simulink subsystem "HEVP3"  (R2024b)
settings: Solver=VariableStepAuto  StartTime=0.0  StopTime=10.0  RelTol=1e-3
undefined symbols (not defined in the file): Diff, Eng, Lock, PlntDriveshftDamp, PlntDriveshftStiff, PlntTransEffTempBpt, PlntTransGearRatioVect, Trans, up
libraries: autolibsharedcoupling x2, autolibsharedtransfixedgear x1, autolibtrqconv x1
settings Model: ModifiedByFormat=The MathWorks, Inc.  Creator=The MathWorks, Inc.  LastModifiedBy=The MathWorks, Inc.
settings SolverCC: MaxZcPerStep=1
settings DebuggingCC: UnconnectedInputMsg=warning  UnconnectedOutputMsg=warning  UnconnectedLineMsg=warning
settings ModelReferenceCC: EnableRefExpFcnMdlSchedulingChecks=on
settings RTWCC: GPUComputeCapability=3.5  DLArmComputeVersion=19.05

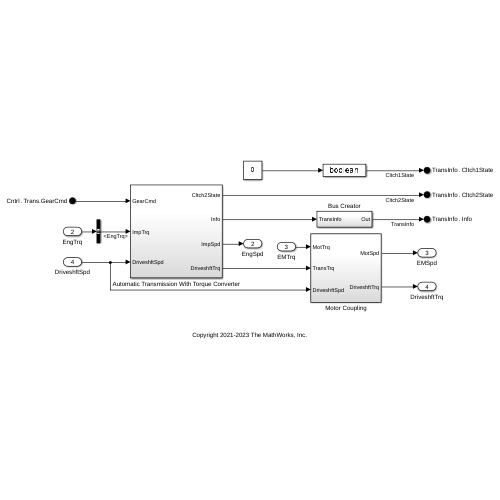
[thumbnail: Simulink's stored preview of the top-level diagram]
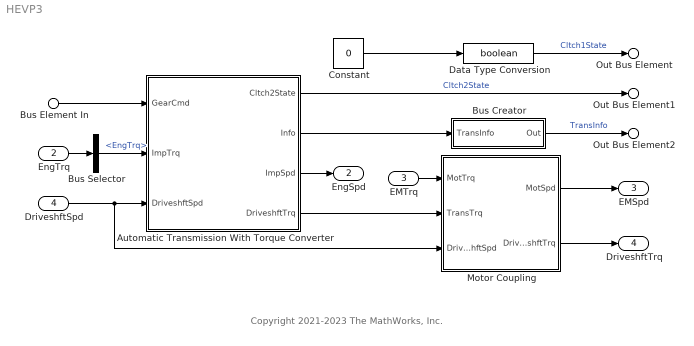
== system HEVP3 ==
  note: Copyright 2021-2023 The MathWorks, Inc.
  Bus Element In : Inport  PortName=Cntrl  Element=Trans.GearCmd
  EngTrq : Inport  Port=2
  EMTrq : Inport  Port=3
  DriveshftSpd : Inport  Port=4
  Automatic Transmission With Torque Converter : Subsystem  VariantControl=1
  Bus Selector : BusSelector  OutputSignals=EngTrq
  Bus Creator : Subsystem
  Constant : Constant  Value=0  SampleTime=-1
  Data Type Conversion : DataTypeConversion  OutDataTypeStr=boolean  SaturateOnIntegerOverflow=off  RndMeth=Floor
  Motor Coupling : Subsystem
  Out Bus Element : Outport  PortName=TransInfo  Element=Cltch1State
  Out Bus Element1 : Outport  PortName=TransInfo  Element=Cltch2State
  Out Bus Element2 : Outport  PortName=TransInfo  Element=Info
  EngSpd : Outport  Port=2  VectorParamsAs1DForOutWhenUnconnected=off  BusOutputAsStruct=on
  EMSpd : Outport  Port=3  VectorParamsAs1DForOutWhenUnconnected=off  BusOutputAsStruct=on
  DriveshftTrq : Outport  Port=4  VectorParamsAs1DForOutWhenUnconnected=off
  wires:
  Motor Coupling/1(MotSpd) -> EMSpd/1
  Bus Element In/1 -> Automatic Transmission With Torque Converter/1(GearCmd)
  EngTrq/1 -> Bus Selector/1
  EMTrq/1 -> Motor Coupling/1(MotTrq)
  Automatic Transmission With Torque Converter/3(ImpSpd) -> EngSpd/1
  DriveshftSpd/1 -> Automatic Transmission With Torque Converter/3(DriveshftSpd), Motor Coupling/3(DriveshftSpd)
  Automatic Transmission With Torque Converter/4(DriveshftTrq) -> Motor Coupling/2(TransTrq)
  Motor Coupling/2(DriveshftTrq) -> DriveshftTrq/1
  Automatic Transmission With Torque Converter/1(Cltch2State) -> Out Bus Element1/1  "Cltch2State"
  Data Type Conversion/1 -> Out Bus Element/1  "Cltch1State"
  Constant/1 -> Data Type Conversion/1
  Bus Selector/1 -> Automatic Transmission With Torque Converter/2(ImpTrq)  "<EngTrq>"
  Bus Creator/1(Out) -> Out Bus Element2/1  "TransInfo"
  Automatic Transmission With Torque Converter/2(Info) -> Bus Creator/1(TransInfo)

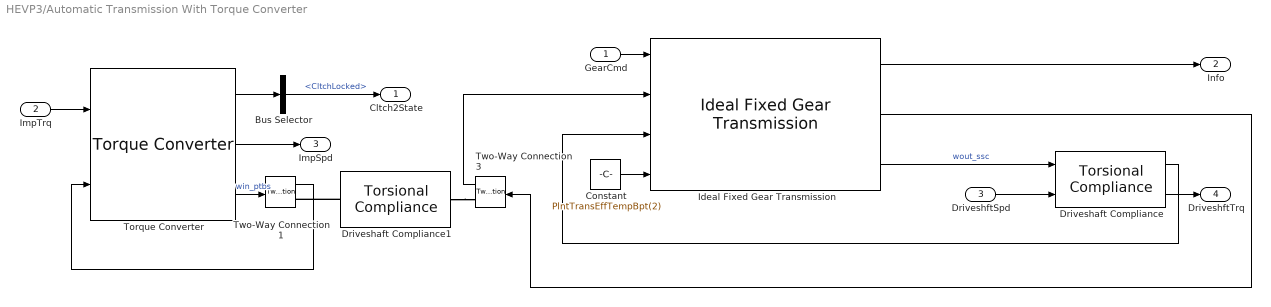
== system HEVP3/Automatic Transmission With Torque Converter ==
  GearCmd : Inport
  ImpTrq : Inport  Port=2
  DriveshftSpd : Inport  Port=3
  Bus Selector : BusSelector  OutputSignals=Cltch.CltchLocked
  Constant : Constant  Value=PlntTransEffTempBpt(2)  SampleTime=-1
  Driveshaft Compliance : autolibsharedcoupling/Torsional Compliance  port_config=Simulink  extInfo=off  k=PlntDriveshftStiff  b=PlntDriveshftDamp  theta_o=PlntDriveshftInitDeflect  domega_o=PlntDriveshftInitVel  omega_c=PlntDriveshftDampCutoffFreq  blkID=0  aMode=1
  Driveshaft Compliance1 : autolibsharedcoupling/Torsional Compliance  port_config=Two-way connection  extInfo=off  k=PlntDriveshftStiff  b=PlntDriveshftDamp  theta_o=PlntDriveshftInitDeflect  domega_o=PlntDriveshftInitVel  omega_c=PlntDriveshftDampCutoffFreq  blkID=0  aMode=1
  Ideal Fixed Gear Transmission : autolibsharedtransfixedgear/Ideal Fixed Gear Transmission  VariantControl=0  TransEffModelPopup=Gear, input torque, input speed, and temperature  gearInterp=Linear point-slope  G=PlntTransGearNumVect  Trq_bpts=PlntTransEffTrqBpt  omega_bpts=PlntTransEffSpdBpt  Temp_bpts=PlntTransEffTempBpt  N=PlntTransGearRatioVect  Jout=PlntTransInertiaVect  bout=PlntTransDampVect  eta=PlntTransEffVect  eta_tbl=PlntTransEffTbl  G_o=PlntTransInitGear  omega_o=PlntTransInitOutVel  omegaN_o=PlntTransInitNtrlInVel  tau_s=PlntTransShftTimeCnst  maxAbsSpd=5e3  aMode=6
  Torque Converter : autolibtrqconv/Torque Converter  TCType=Lock-up  port_config=Simulink  Ji=PlntTrqConvrtrImpInertia  bi=PlntTrqConvrtrImpDamp  Jt=PlntTrqConvrtrTurbInertia  bt=PlntTrqConvrtrTurbDamp  omegai_o=PlntTrqConvrtrImpInitVel  omegat_o=PlntTrqConvrtrTurbInitVel  phi=PlntTrqConvrtrSpdRatioVect  KType=Input speed / sqrt(input torque)  psi=PlntTrqConvrtrCapVect  zeta=PlntTrqConvrtrTrqRatioVect  tauTC=PlntTrqConvrtrTimeCnst  InterpMethod=Linear  Reff=PlntTrqConvrtrCltchRadius  mus=PlntTrqConvrtrCltchStatFric  muk=PlntTrqConvrtrCltchKinFric  ClutchLocked=off  philu=PlntTrqConvrtrCltchLckUpSpdRatio  omegal=PlntTrqConvrtrCltchMinLckUpEngdSpd  omegau=PlntTrqConvrtrCltchMinLckUpDisengdSpd  K_c=PlntTrqConvrtrCltchLckUpForceGain  tauC=PlntTrqConvrtrCltchLckUpTimeCnst  maxAbsSpd=5e3  tau_dl=3000
      settings: AttributesFormatString="Lock-up type:  %<TCType>"
  Two-Way Connection1 : TwoWayConnection
  Two-Way Connection3 : TwoWayConnection
  Cltch2State : Outport  VectorParamsAs1DForOutWhenUnconnected=off
  Info : Outport  Port=2  VectorParamsAs1DForOutWhenUnconnected=off
  ImpSpd : Outport  Port=3  VectorParamsAs1DForOutWhenUnconnected=off
  DriveshftTrq : Outport  Port=4  VectorParamsAs1DForOutWhenUnconnected=off
  wires:
  DriveshftSpd/1 -> Driveshaft Compliance/2
  Torque Converter/3 -> Two-Way Connection1/1  "win_ptbs"
  Two-Way Connection3/1 -> Ideal Fixed Gear Transmission/2
  Torque Converter/2 -> ImpSpd/1
  ImpTrq/1 -> Torque Converter/1
  GearCmd/1 -> Ideal Fixed Gear Transmission/1
  Ideal Fixed Gear Transmission/1 -> Info/1
  Torque Converter/1 -> Bus Selector/1
  Ideal Fixed Gear Transmission/2 -> Two-Way Connection3/1
  Driveshaft Compliance/1 -> Ideal Fixed Gear Transmission/3
  Two-Way Connection1/1 -> Torque Converter/2
  Ideal Fixed Gear Transmission/3 -> Driveshaft Compliance/1  "wout_ssc"
  Bus Selector/1 -> Cltch2State/1  "<CltchLocked>"
  Constant/1 -> Ideal Fixed Gear Transmission/4
  Driveshaft Compliance/2 -> DriveshftTrq/1
  connections:
  Driveshaft Compliance1/RConn1 -- Two-Way Connection3/RConn1
  Driveshaft Compliance1/LConn1 -- Two-Way Connection1/RConn1

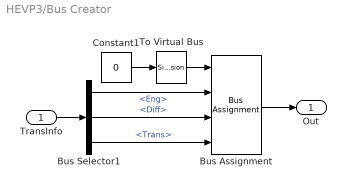
== system HEVP3/Bus Creator ==
  TransInfo : Inport
  Bus Assignment : BusAssignment  AssignedSignals=Eng,Diff,Trans
  Bus Selector1 : BusSelector  OutputSignals=Eng,Diff,Trans
  Constant1 : Constant  Value=0  OutDataTypeStr=Bus: InfoBUS  SampleTime=Inf
  To Virtual Bus : SignalConversion  ConversionOutput=Virtual bus  OverrideOpt=off
  Out : Outport
  wires:
  To Virtual Bus/1 -> Bus Assignment/1
  Constant1/1 -> To Virtual Bus/1
  TransInfo/1 -> Bus Selector1/1
  Bus Selector1/3 -> Bus Assignment/4  "<Trans>"
  Bus Selector1/1 -> Bus Assignment/2  "<Eng>"
  Bus Selector1/2 -> Bus Assignment/3  "<Diff>"
  Bus Assignment/1 -> Out/1

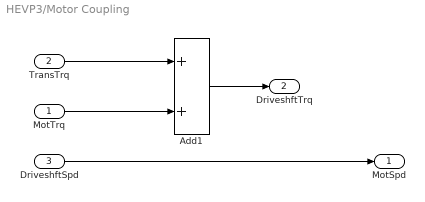
== system HEVP3/Motor Coupling ==
  MotTrq : Inport
  TransTrq : Inport  Port=2
  DriveshftSpd : Inport  Port=3
  Add1 : Sum
  MotSpd : Outport  VectorParamsAs1DForOutWhenUnconnected=off  BusOutputAsStruct=on
  DriveshftTrq : Outport  Port=2  VectorParamsAs1DForOutWhenUnconnected=off
  wires:
  DriveshftSpd/1 -> MotSpd/1
  Add1/1 -> DriveshftTrq/1
  TransTrq/1 -> Add1/1
  MotTrq/1 -> Add1/2
